simulink model "cars"  (R2022b)
settings: Solver=FixedStepAuto  StartTime=0  StopTime=timeFinal  FixedStep=timeStepMax  MinStep=0.01  RelTol=1e-3  AbsTol=1e-5  EnableMultiTasking=on
settings Model: Creator=yoriyuki  LastModifiedBy=jun
settings SolverCC: AlgebraicLoopSolver=TrustRegion  AutoInsertRateTranBlk=on
settings DataIOCC: ExternalInput=[Throttle, Brake]  FinalStateName=SavePoint  InitialState=SavePoint  SaveOperatingPoint=on  SaveOutput=off  SaveTime=off  ReturnWorkspaceOutputs=off  StateSaveName=x  TimeSaveName=t  OutputSaveName=y
settings OptimizationCC: LifeSpan=inf
settings DebuggingCC: UnconnectedInputMsg=warning  UnconnectedOutputMsg=warning  UnconnectedLineMsg=warning  AllowSymbolicDim=off  SFUnexpectedBacktrackingDiag=warning  SFNoUnconditionalDefaultTransitionDiag=warning  SFExecutionAtInitializationDiag=none  SFMachineParentedDataDiag=warning  ArithmeticOperatorsInVariantConditions=warning
settings ModelReferenceCC: EnableRefExpFcnMdlSchedulingChecks=on
settings SFSimCC: SimUseLocalCustomCode=off  CustomCodeUndefinedFunction=UseInterfaceOnly
settings RTWCC: RTWUseLocalCustomCode=off
settings CodeAppCC: StateflowObjectComments=on
settings GRTTargetCC: TargetLangStandard=C89/C90 (ANSI)
settings ConfigComp: CovMetricSettings=dw  CovSaveCumulativeToWorkspaceVar=on  CovSaveSingleToWorkspaceVar=on  CovExternalEMLEnable=off

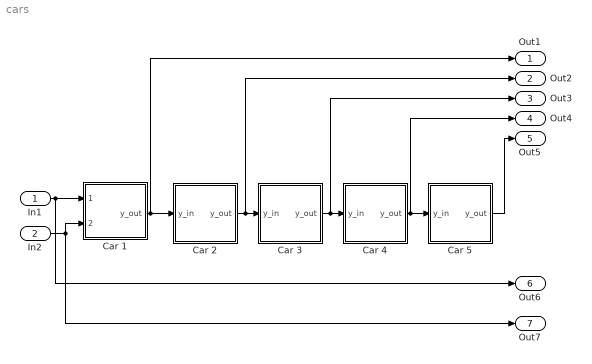
== system cars ==
  In1 : Inport
  In2 : Inport  Port=2
  Car 1 : Stateflow chart  TreatAsAtomicUnit=on
  Car 2 : Stateflow chart  TreatAsAtomicUnit=on
  Car 3 : Stateflow chart  TreatAsAtomicUnit=on
  Car 4 : Stateflow chart  TreatAsAtomicUnit=on
  Car 5 : Stateflow chart  TreatAsAtomicUnit=on
  Out1 : Outport  VectorParamsAs1DForOutWhenUnconnected=off
  Out2 : Outport  Port=2  VectorParamsAs1DForOutWhenUnconnected=off
  Out3 : Outport  Port=3  VectorParamsAs1DForOutWhenUnconnected=off
  Out4 : Outport  Port=4  VectorParamsAs1DForOutWhenUnconnected=off
  Out5 : Outport  Port=5  VectorParamsAs1DForOutWhenUnconnected=off
  Out6 : Outport  Port=6
  Out7 : Outport  Port=7
  wires:
  Car 5/1(y_out) -> Out5/1
  Car 1/1(y_out) -> Out1/1, Car 2/1(y_in)
  Car 2/1(y_out) -> Out2/1, Car 3/1(y_in)
  Car 3/1(y_out) -> Out3/1, Car 4/1(y_in)
  Car 4/1(y_out) -> Car 5/1(y_in), Out4/1
  In1/1 -> Out6/1, Car 1/1(Throttle)
  In2/1 -> Car 1/2(Brake), Out7/1

== stateflow chart cars/Car 1 ==
  settings: updateMethod=CONTINUOUS
  state Run
    during:
    v_dot = -Throttle - Brake * v;
    y_dot = v;
    y_out = y;
  (default) -> Run
  data: Throttle input; Brake input; y local =0; y_out output; v local =0
  data y settings: updateMethod=SF_CONTINUOUS_TIME_DATA
  data v settings: updateMethod=SF_CONTINUOUS_TIME_DATA

== stateflow chart cars/Car 3 ==
  settings: updateMethod=CONTINUOUS
  state Chasing
    during:
    v_dot = 1;
    y_dot = -v;
    y_out = y;
  state Keeping
    during:
    y_dot = v;
    y_out = y;
  state Braking
    during:
    v_dot = -v;
    y_dot = -v;
    y_out = y;
  (default) -> Keeping
  Chasing -> Keeping : [y - y_in <= 10]
      | % [transition condition]{action}
  Keeping -> Chasing [order 1] : [y - y_in >=15]
  Braking -> Chasing : [y - y_in >= 20]
  Keeping -> Braking [order 2] : [y - y_in <=5]
  data: y_out output; y local double =20; v local =0; y_in input
  data y settings: updateMethod=SF_CONTINUOUS_TIME_DATA
  data v settings: updateMethod=SF_CONTINUOUS_TIME_DATA
  data y_in settings: updateMethod=SF_CONTINUOUS_TIME_DATA

== stateflow chart cars/Car 2 ==
  settings: updateMethod=CONTINUOUS
  state Chasing
    during:
    v_dot = 1;
    y_dot = -v;
    y_out = y;
  state Keeping
    during:
    y_dot = v;
    y_out = y;
  state Braking
    during:
    v_dot = -v;
    y_dot = -v;
    y_out = y;
  (default) -> Keeping
  Chasing -> Keeping : [y - y_in <= 10]
  Keeping -> Chasing [order 1] : [y - y_in >=15]
  Braking -> Chasing : [y - y_in >= 20]
  Keeping -> Braking [order 2] : [y - y_in <=5]
  data: y_out output; y local double =10; v local =0; y_in input
  data y settings: updateMethod=SF_CONTINUOUS_TIME_DATA
  data v settings: updateMethod=SF_CONTINUOUS_TIME_DATA
  data y_in settings: updateMethod=SF_CONTINUOUS_TIME_DATA

== stateflow chart cars/Car 4 ==
  settings: updateMethod=CONTINUOUS
  state Chasing
    during:
    v_dot = 1;
    y_dot = -v;
    y_out = y;
  state Keeping
    during:
    y_dot = v;
    y_out = y;
  state Braking
    during:
    v_dot = -v;
    y_dot = -v;
    y_out = y;
  (default) -> Keeping
  Chasing -> Keeping : [y - y_in <= 10]
      | % [transition condition]{action}
  Keeping -> Chasing [order 1] : [y - y_in >=15]
  Braking -> Chasing : [y - y_in >= 20]
  Keeping -> Braking [order 2] : [y - y_in <=5]
  data: y local double =30; v local =0; y_in input; y_out output
  data y settings: updateMethod=SF_CONTINUOUS_TIME_DATA
  data v settings: updateMethod=SF_CONTINUOUS_TIME_DATA
  data y_in settings: updateMethod=SF_CONTINUOUS_TIME_DATA

== stateflow chart cars/Car 5 ==
  settings: updateMethod=CONTINUOUS
  state Keeping
    during:
    y_dot = v;
    y_out = y;
  state Chasing
    during:
    v_dot = 1;
    y_dot = -v;
    y_out = y;
  state Braking
    during:
    v_dot = -v;
    y_dot = -v;
    y_out = y;
  (default) -> Keeping
  Chasing -> Keeping : [y - y_in <= 10]
      | % [transition condition]{action}
  Keeping -> Chasing [order 1] : [y - y_in >=15]
  Braking -> Chasing : [y - y_in >= 20]
  Keeping -> Braking [order 2] : [y - y_in <=5]
  data: y_out output; y local double =40; v local =0; y_in input
  data y settings: updateMethod=SF_CONTINUOUS_TIME_DATA
  data v settings: updateMethod=SF_CONTINUOUS_TIME_DATA
  data y_in settings: updateMethod=SF_CONTINUOUS_TIME_DATA
